simulink model "DrTekes_Lab6Model"  (R2016a)
settings: Solver=ode4  StartTime=0.0  StopTime=10.0  FixedStep=0.001  RelTol=1e-3
libraries: powerlib_meascontrol x3
settings Model: Creator=atekes  LastModifiedBy=atekes

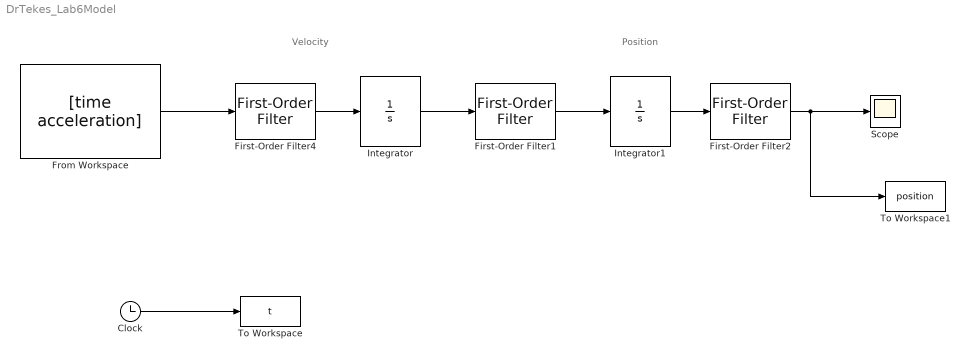
== system DrTekes_Lab6Model ==
  note: Position
  note: Velocity
  Clock : Clock
  First-Order Filter1 : powerlib_meascontrol/Filters/First-Order Filter  FilterType=Highpass  Tc=1  Ts=0  Initialize=on  Vac_Init=[0, 0, 100]  Vdc_Init=0  PlotResponse=off  FreqRange="[0,  200,  1]"
  First-Order Filter2 : powerlib_meascontrol/Filters/First-Order Filter  FilterType=Highpass  Tc=1  Ts=0  Initialize=on  Vac_Init=[0, 0, 100]  Vdc_Init=0  PlotResponse=off  FreqRange="[0,  200,  1]"
  First-Order Filter4 : powerlib_meascontrol/Filters/First-Order Filter  FilterType=Highpass  Tc=1  Ts=0  Initialize=on  Vac_Init=[0, 0, 100]  Vdc_Init=0  PlotResponse=off  FreqRange="[0,  200,  1]"
  From Workspace : FromWorkspace  VariableName=[time acceleration]  SampleTime=0.001  OutputAfterFinalValue=Setting to zero
  Integrator : Integrator
  Integrator1 : Integrator  InitialCondition=3/100  LimitOutput=on  UpperSaturationLimit=3/100  LowerSaturationLimit=-3/100
  Scope : Scope
  To Workspace : ToWorkspace  VariableName=t  SampleTime=-1
  To Workspace1 : ToWorkspace  VariableName=position  SampleTime=-1
  wires:
  From Workspace/1 -> First-Order Filter4/1
  Integrator/1 -> First-Order Filter1/1
  Integrator1/1 -> First-Order Filter2/1
  First-Order Filter4/1 -> Integrator/1
  First-Order Filter1/1 -> Integrator1/1
  First-Order Filter2/1 -> To Workspace1/1, Scope/1
  Clock/1 -> To Workspace/1
